simulink model "L_12_05_21_effetti_sul_comando_schema"  (R2021a)
settings: Solver=VariableStepAuto  StartTime=0.0  StopTime=10.0  RelTol=1e-3
libraries: cstblocks x2
settings Model: Creator=armandofornasier  LastModifiedBy=armandofornasier

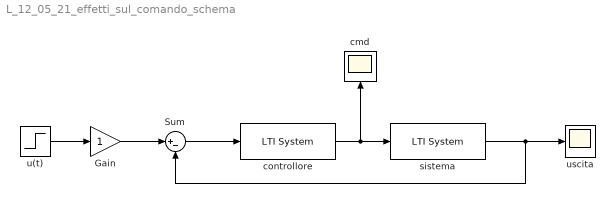
== system L_12_05_21_effetti_sul_comando_schema ==
  Gain : Gain
  Sum : Sum  Inputs=|+-
  cmd : Scope
  controllore : cstblocks/LTI System  sys=C  IC=[]
  sistema : cstblocks/LTI System  sys=F  IC=[]
  u(t) : Step  Time=0  SampleTime=0
  uscita : Scope
  wires:
  u(t)/1 -> Gain/1
  Gain/1 -> Sum/1
  Sum/1 -> controllore/1
  controllore/1 -> cmd/1, sistema/1
  sistema/1 -> uscita/1, Sum/2
